simulink model "NLADRC2"  (R2023a)
settings: Solver=VariableStepAuto  StartTime=0.0  StopTime=10  RelTol=1e-3
settings Model: Creator=belov  LastModifiedBy=belov

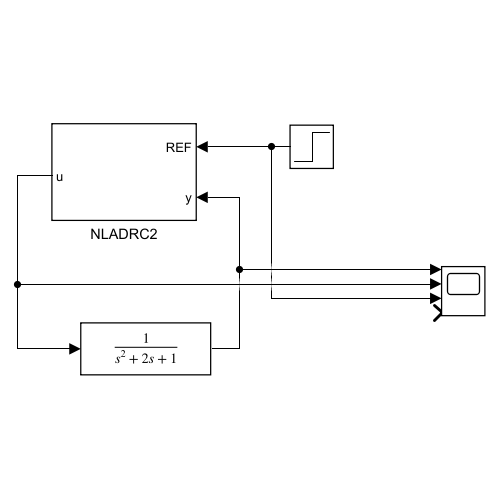
[thumbnail: Simulink's stored preview of the top-level diagram]
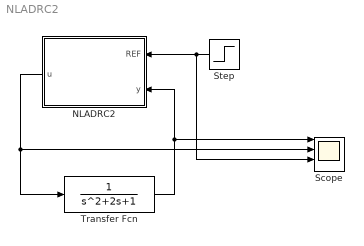
== system NLADRC2 ==
  NLADRC2 : Subsystem
  Scope : Scope  NumInputPorts=4
  Step : Step  SampleTime=0.001
  Transfer Fcn : TransferFcn
  wires:
  Transfer Fcn/1 -> Scope/1, NLADRC2/2(y)
  NLADRC2/1(u) -> Transfer Fcn/1, Scope/2
  Step/1 -> NLADRC2/1(REF), Scope/3

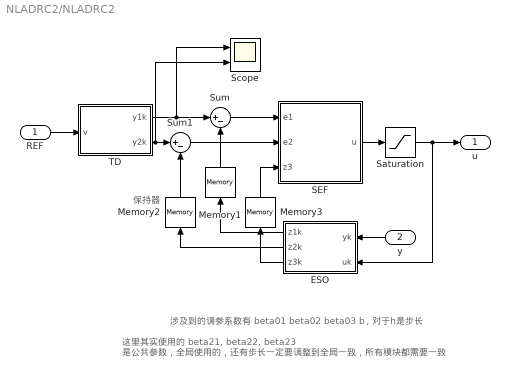
== system NLADRC2/NLADRC2 ==
  note: 这里其实使用的 beta21, beta22, beta23 是公共参数，全局使用的，还有步长一定要调整到全局一致，所有模块都需要一致
  note: 保持器
  note: 涉及到的调参系数有 beta01 beta02 beta03 b，对于h是步长
  REF : Inport
  y : Inport  Port=2
  ESO : MATLAB Function  TreatAsAtomicUnit=on  SystemSampleTime=0.001
  Memory1 : Memory
  Memory2 : Memory
  Memory3 : Memory
  SEF : MATLAB Function  TreatAsAtomicUnit=on  SystemSampleTime=0.001
  Saturation : Saturate  UpperLimit=10  LowerLimit=-10
  Scope : Scope  NumInputPorts=2
  Sum : Sum  Inputs=|+-
  Sum1 : Sum  Inputs=|+-
  TD : MATLAB Function  TreatAsAtomicUnit=on  SystemSampleTime=0.001
  u : Outport
  wires:
  ESO/1(z1k) -> Memory1/1
  ESO/2(z2k) -> Memory2/1
  Memory1/1 -> Sum/2
  Sum/1 -> SEF/1(e1)
  ESO/3(z3k) -> Memory3/1
  TD/1(y1k) -> Scope/1, Sum/1
  REF/1 -> TD/1(v)
  TD/2(y2k) -> Scope/2, Sum1/1
  Memory2/1 -> Sum1/2
  y/1 -> ESO/1(yk)
  Memory3/1 -> SEF/3(z3)
  SEF/1(u) -> Saturation/1
  Saturation/1 -> u/1, ESO/2(uk)
  Sum1/1 -> SEF/2(e2)

== matlab function NLADRC2/TD ==
  data: v input; y1k output; y2k output
function [y1k,y2k] = TD(v)

persistent y1k_1 y2k_1

if isempty(y1k_1)
    y1k_1 = 0;
end
if isempty(y2k_1)
    y2k_1 = 0;
end

h = 0.001; % 步长
r = 10; % 但是实际上r过大反而会导致系统更慢趋近于平稳

%%%% 这是一种 TD 的形式
% Filterfactor = 0.01; % 滤波因子
% e1 = y1k_1 - v; % 期望之差
% 
% %%%% hst 解算
% d = r * Filterfactor;
% d0 = Filterfactor * d;
% y = y1k_1 + Filterfactor * y2k_1 - v;
% a0 = sqrt(d^2 + 8 * r * abs(y));
% a = 0;
% fst = 0;
% if abs(y) > d0
%     a = y2k_1 + (a0 - d) / 2 * sign(y);
% else
%     a = y2k_1 + y / Filterfactor;
% end
% if abs(a) > d
%     fst = -r * sign(a);
% else
%     fst = -r * a / d;
% end
% 
% y1k = y1k_1 + h * y2k_1;
% y2k = y2k_1 + h * fst;

%%%% 这又是一种TD的形式，效果还是挺不错的
y1k = y1k_1 + h * y2k_1;
y2k = y2k_1 + h * (-r * r * (y1k_1 - v) - 2 * r * y2k_1);

%%%% 第三种TD方式 
%%%% fhan解算
% h1 = 0.01;
% d = r * h1 * h1;
% a0 = h1 * y2k_1;
% y = y1k_1 - v + a0;
% a1 = sqrt(d * (d + 8 * abs(y)));
% a2 = a0 + (a1 - d) / 2 * sign(y);
% fsgyd = (sign(y + d) - sign(y - d)) / 2;
% a = (a0 + y) * fsgyd + a2 * (1 - fsgyd);
% fsgad = (sign(a + d) - sign(a - d)) / 2;
% fhan = -r * a / d * fsgad - r * sign(a) * (1 - fsgad);
% 
% y1k = y1k_1 + h * y2k_1;
% y2k = y2k_1 + h * fhan;

y1k_1 = y1k;
y2k_1 = y2k;
end

== matlab function NLADRC2/SEF ==
  data: e1 input; u output; e2 input; z3 input
function u =SEF(e1,e2,z3)
%%%% 一共有四种非线性反馈控制率 就是4种u0的控制率
%%%% 第一种 效果很好
h = 0.001; % 步长
b0 = 6;
beta1=1000;
beta2=200;
u0 = beta1 * e1 + beta2 * e2;
u = u0 - z3 / b0;
u = u * b0;

%%%% 第二种 实际上最后的输出结果还算不错
% alfa1=0.99;
% alfa2=0.99;
% delta=0.002;
% beta1=1000;
% beta2=200;
% fal1=1;
% fal2=1;
% 
% if abs(e1)<=delta
%     fal1=e1/(delta^(1-alfa1));
% else
%     fal1=(abs(e1))^(alfa1)*sign(e1);
% end
% 
% if abs(e2)<=delta
%     fal2=e2/(delta^(1-alfa2));
% else
%     fal2=(abs(e2))^(alfa2)*sign(e2);
% end
% 
% u0=beta1*fal1+beta2*fal2;
% b0 = 1;
% u = u0 - z3 / b0;
% u = u * b0;


%%%% 第三种 感觉很方便，但是效果不是很好，会把处理出来的 u 产生高频震荡，需要调节参数，我真的是麻了
%%%% 其实就是需要将 z3 项放大来抵消 e1 e2 项所导致的高频振荡，但是太抽象了
%%%% fhan(e1, e2, r, h) 个人认为这里的r 应该和TD里面的r一致的 这里的b0应该与ESO中的b0一致
% h = 0.001; % 步长
% r = 1000;
% b0 = 0.01;
% Filterfactor = 0.02; % 滤波因子
% d = r * h * h;
% a0 = Filterfactor * e2;
% y = e1 + a0;
% a1 = sqrt(d * (d + 8 * abs(y)));
% a2 = a0 + (a1 - d) / 2 * sign(y);
% fsgyd = (sign(y + d) - sign(y - d)) / 2;
% a = (a0 + y) * fsgyd + a2 * (1 - fsgyd);
% fsgad = (sign(a + d) - sign(a - d)) / 2;
% fhan = -r * a / d * fsgad - r * sign(a) * (1 - fsgad);
% 
% u0 = -fhan;
% u = u0 - z3 / b0;
% u = u * b0;

% %%%% 第四种，也就是e2处加了个系数而已 跟第三种差不多吧
% c = 1; % 系数可调吧....但是调不了一点
% e2 = c * e2;
% h = 0.001; % 步长
% r = 1000;
% b0 = 0.01;
% Filterfactor = 0.02; % 滤波因子
% d = r * h * h;
% a0 = Filterfactor * e2;
% y = e1 + a0;
% a1 = sqrt(d * (d + 8 * abs(y)));
% a2 = a0 + (a1 - d) / 2 * sign(y);
% fsgyd = (sign(y + d) - sign(y - d)) / 2;
% a = (a0 + y) * fsgyd + a2 * (1 - fsgyd);
% fsgad = (sign(a + d) - sign(a - d)) / 2;
% fhan = -r * a / d * fsgad - r * sign(a) * (1 - fsgad);
% 
% u0 = -fhan;
% u = u0 - z3 / b0;
% u = u * b0;

end

== matlab function NLADRC2/ESO ==
  settings: updateMethod=DISCRETE  sampleTime=0.001
  data: yk input; z1k output; uk input; z2k output; z3k output
function [z1k,z2k,z3k] = ESO(yk,uk)
persistent z1k_1 z2k_1 z3k_1

h = 0.001; % 步长
wc = 5; % 带宽 需要调节
wo = 3 * wc;

beta21 = 3 * wo;
beta22 = 3 * wo * wo;
beta23 = wo ^ 3;

b0 = 1;

alpha2 = 1;
delta2 = 0.002; % 2h

alpha3 = 1;
delta3 = 0.002;

if isempty(z1k_1)
    z1k_1 = 0;
end
if isempty(z2k_1)
    z2k_1 = 0;
end
if isempty(z3k_1)
    z3k_1 = 0;
end

e2 = z1k_1 - yk;

%%%% fal计算
e2abs = abs(e2);
fal2 = 0;
if e2abs <= delta2
    fal2 = e2abs ^ alpha2 * sign(e2);
else 
    fal2 = e2 / (delta2 ^ (1 - alpha2));
end
fal3 = 0;
if e2abs <= delta3
    fal3 = e2abs ^ alpha3 * sign(e2);
else 
    fal3 = e2 / (delta3 ^ (1 - alpha3));
end

z1k = h * (z2k_1 - beta21 * e2) + z1k_1;
z2k = h * (z3k_1 - beta22 * fal2 + b0 * uk) + z2k_1;
z3k = h * (-beta23 * fal3) + z3k_1;

z1k_1 = z1k;
z2k_1 = z2k;
z3k_1 = z3k;

end
